simulink model "ESP_ABS"  (R2020b)
settings: Solver=VariableStepAuto  StartTime=0.0  StopTime=5  RelTol=1e-3
InitFcn:
  | ABS_F = 'ABS';
  | ABS_R = 'ABS';
  | ESP = 'ESP_moment2'
  | 
  | a = 1.203;
  | b = 1.217;
  | L = a + b;
libraries: fuzblock x5, simulink x1
settings Model: SimulationMode=accelerator  Creator=hadlaczkyb  LastModifiedBy=hadlaczkyb
settings SolverCC: AlgebraicLoopSolver=LineSearch
settings DataIOCC: ReturnWorkspaceOutputs=off
settings OptimizationCC: EfficientMapNaN2IntZero=off
settings DebuggingCC: ArithmeticOperatorsInVariantConditions=warning
settings HardwareCC: TargetBitPerPointer=64  TargetBitPerSizeT=64  TargetBitPerPtrDiffT=64  TargetLongLongMode=on  TargetIntDivRoundTo=Zero  TargetEndianess=LittleEndian  TargetWordSize=64  TargetHWDeviceType=MATLAB Host  ProdEqTarget=off
settings SFSimCC: SimUseLocalCustomCode=off  CustomCodeUndefinedFunction=UseInterfaceOnly
settings RTWCC: RTWUseLocalCustomCode=off
settings CodeAppCC: MaxIdLength=128
settings GRTTargetCC: TargetLangStandard=C89/C90 (ANSI)  CombineOutputUpdateFcns=off  GRTInterface=on

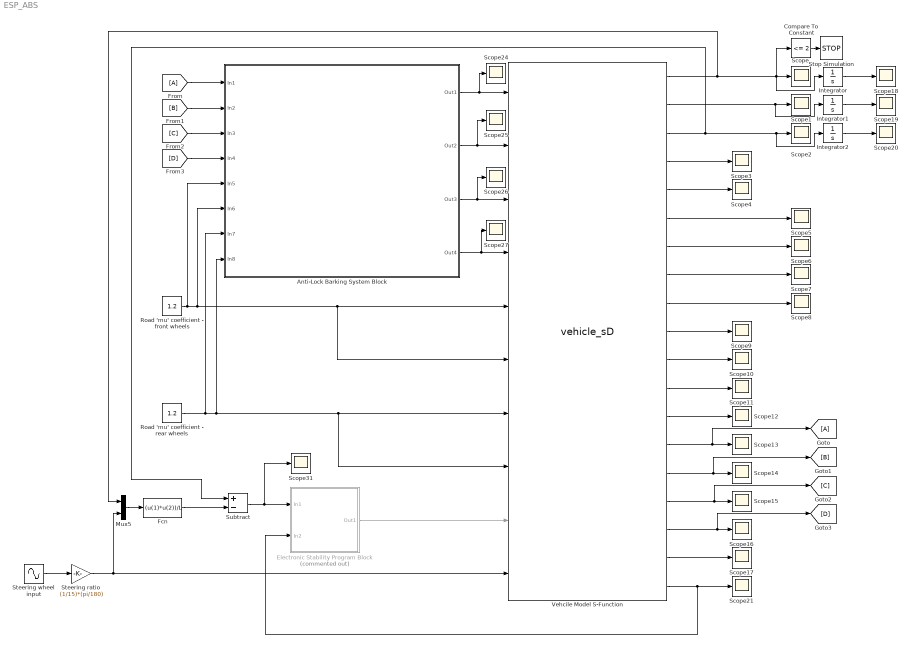
== system ESP_ABS ==
  Anti-Lock Barking System Block : Subsystem
      mask Display:
      | image('Fuzzy_ABS_ESP/ABS_icon.png');
      | port_label('input',1,'\sigma_{FL}','texmode','on');
      | port_label('input',2,'\sigma_{FR}','texmode','on');
      | port_label('input',3,'\sigma_{RL}','texmode','on');
      | port_label('input',4,'\sigma_{RR}','texmode','on');
      | port_label('input',5,'\mu_{FL}','texmode','on');
      | port_label('input',6,'\mu_{FR}','texmode','on');
      | port_label('input',7,'\mu_{RL}','texmode','on');
      | port_label('input',8,'\mu_{RR}','texmode','on');
      | port_label('output',1,'Tb_{FL}','texmode','on');
      | port_label('output',2,'Tb_{FR}','texmode','on');
      | port_label('output',3,'Tb_{RL}','texmode','on');
      | port_label('output',4,'Tb_{RR}','texmode','on');
  Compare To Constant : simulink/Logic and Bit Operations/Compare To Constant  relop=<=  const=2  OutDataTypeStr=boolean
  Electronic Stability Program Block : Subsystem  Commented=on
      mask Display:
      | image('Fuzzy_ABS_ESP/ESP_icon.png');
      | port_label('input',1,'\psi_e','texmode','on');
      | port_label('input',2,'\beta_e','texmode','on');
      | port_label('output',1,'M_z','texmode','on');
  Fcn : Fcn  Expr=(u(1)*u(2))/L
      mask Display: disp('\psi_d','texmode','on');
  Integrator : Integrator
  Integrator1 : Integrator
  Integrator2 : Integrator
  Mux5 : Mux  Inputs=2
  Road 'mu' coefficient - front wheels : Constant  Value=1.2
  Road 'mu' coefficient - rear wheels : Constant  Value=1.2
  Scope{,1..21,24..27,31} (27 alike) : Scope
  Steering ratio : Gain  Gain=(1/15)*(pi/180)
  Steering wheel input : Sin  Amplitude=0  Frequency=(2*pi)/5  SampleTime=0
  Stop Simulation : Stop
  Subtract : Sum  Inputs=+-
  Vehcile Model S-Function : M-S-Function  FunctionName=vehicle_sD
      mask Display:
      | disp('Full vehicle model');
      | port_label('input',1, 'Tb_{FL}','texmode','on');
      | port_label('input',2, 'Tb_{FR}','texmode','on');
      | port_label('input',3, 'Tb_{RL}','texmode','on');
      | port_label('input',4, 'Tb_{RR}','texmode','on');
      | port_label('input',5, '\mu_{FL}','texmode','on');
      | port_label('input',6, '\mu_{FR}','texmode','on');
      | port_label('input',7, '\mu_{RL}','texmode','on');
      | port_label('input',8, '\mu_{RR}','texmode','on');
      | port_label('input',9, 'M_z','texmode','on');
      | port_label('input',10, '\delta','texmode','on');
      | port_label('output',1,'v_{vx}','texmode','on');
      | port_label('output',2,'v_{vy}','texmode','on');
      | port_label('output',3,'\psi','texmode','on');
      | port_label('output',4,'a_{vx}','texmode','on');
      | port_label('output',5,'a_{vy}','texmode','on');
      | port_label('output',6,'v_{wxFL}','texmode','on');
      | port_label('output',7,'v_{wxFR}','texmode','on');
      | port_label('output',8,'v_{wxRL}','texmode','on');
      | port_label('output',9,'v_{wxRR}','texmode','on');
      | port_label('output',10,'\omega_{FL}','texmode','on');
      | port_label('output',11,'\omega_{FR}','texmode','on');
      | port_label('output',12,'\omega_{RL}','texmode','on');
      | port_label('output',13,'\omega_{RR}','texmode','on');
      | port_label('output',14,'\sigma_{FL}','texmode','on');
      | port_label('output',15,'\sigma_{FR}','texmode','on');
      | port_label('output',16,'\sigma_{RL}','texmode','on');
      | port_label('output',17,'\sigma_{RR}','texmode','on');
      | port_label('output',18,'v_v','texmode','on');
      | port_label('output',19,'\beta','texmode','on');
  wires:
  Vehcile Model S-Function/2 -> Integrator1/1, Scope1/1
  Vehcile Model S-Function/6 -> Scope5/1
  Vehcile Model S-Function/7 -> Scope6/1
  Vehcile Model S-Function/8 -> Scope7/1
  Vehcile Model S-Function/9 -> Scope8/1
  Vehcile Model S-Function/10 -> Scope9/1
  Vehcile Model S-Function/11 -> Scope10/1
  Vehcile Model S-Function/12 -> Scope11/1
  Vehcile Model S-Function/13 -> Scope12/1
  Vehcile Model S-Function/4 -> Scope3/1
  Vehcile Model S-Function/5 -> Scope4/1
  Integrator/1 -> Scope18/1
  Integrator1/1 -> Scope19/1
  Integrator2/1 -> Scope20/1
  Vehcile Model S-Function/18 -> Scope17/1
  Compare To Constant/1 -> Stop Simulation/1
  Fcn/1 -> Subtract/2
  Mux5/1 -> Fcn/1
  Vehcile Model S-Function/1 -> Mux5/1, Compare To Constant/1, Integrator/1, Scope/1
  Vehcile Model S-Function/15 -> [B], Scope14/1
  Vehcile Model S-Function/17 -> [D], Scope16/1
  Steering wheel input/1 -> Steering ratio/1
  Vehcile Model S-Function/3 -> Subtract/1, Scope2/1, Integrator2/1
  Vehcile Model S-Function/19 -> Electronic Stability Program Block/2(In2), Scope21/1
  Subtract/1 -> Electronic Stability Program Block/1(In1), Scope31/1
  Steering ratio/1 -> Mux5/2, Vehcile Model S-Function/10
  Anti-Lock Barking System Block/4(Out4) -> Scope27/1, Vehcile Model S-Function/4
  Anti-Lock Barking System Block/3(Out3) -> Scope26/1, Vehcile Model S-Function/3
  Anti-Lock Barking System Block/2(Out2) -> Scope25/1, Vehcile Model S-Function/2
  Anti-Lock Barking System Block/1(Out1) -> Scope24/1, Vehcile Model S-Function/1
  [A] -> Anti-Lock Barking System Block/1(In1)
  [B] -> Anti-Lock Barking System Block/2(In2)
  [C] -> Anti-Lock Barking System Block/3(In3)
  [D] -> Anti-Lock Barking System Block/4(In4)
  Electronic Stability Program Block/1(Out1) -> Vehcile Model S-Function/9
  Vehcile Model S-Function/14 -> Scope13/1, [A]
  Vehcile Model S-Function/16 -> Scope15/1, [C]
  Road 'mu' coefficient - front wheels/1 -> Anti-Lock Barking System Block/5(In5), Anti-Lock Barking System Block/6(In6), Vehcile Model S-Function/5, Vehcile Model S-Function/6
  Road 'mu' coefficient - rear wheels/1 -> Anti-Lock Barking System Block/7(In7), Anti-Lock Barking System Block/8(In8), Vehcile Model S-Function/8, Vehcile Model S-Function/7

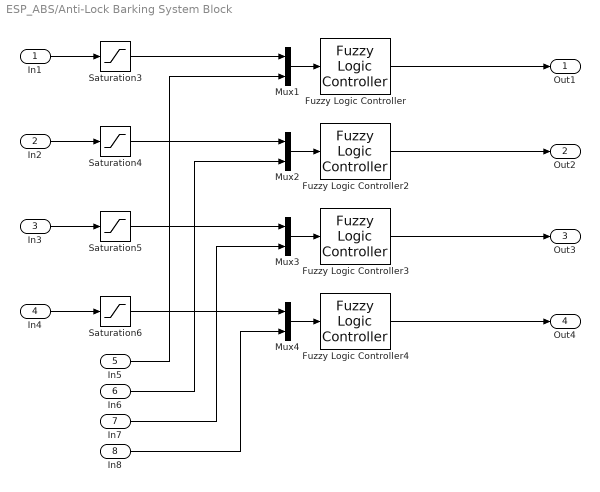
== system ESP_ABS/Anti-Lock Barking System Block ==
  In1 : Inport
  In2 : Inport  Port=2
  In3 : Inport  Port=3
  In4 : Inport  Port=4
  In5 : Inport  Port=5
  In6 : Inport  Port=6
  In7 : Inport  Port=7
  In8 : Inport  Port=8
  Fuzzy Logic Controller{,2..4} (4 alike) : fuzblock/Fuzzy Logic  Controller  FIS=ABS  OutputSampleNumber=101  DataType=double  FuzzifiedInputs=off  RuleFiringStrengths=off  RuleOutputs=off  AggregatedOutputs=off  SimulateUsing=Interpreted execution  OutOfRangeInputValueMessage=warning  NoRuleFiredMessage=warning  EmptyOutputFuzzySetMessage=warning
  Mux{1..4} (4 alike) : Mux  Inputs=2
  Saturation3 : Saturate  UpperLimit=0.15  LowerLimit=0.06
  Saturation4 : Saturate  UpperLimit=0.15  LowerLimit=0.06
  Saturation5 : Saturate  UpperLimit=0.14  LowerLimit=0.055
  Saturation6 : Saturate  UpperLimit=0.14  LowerLimit=0.055
  Out1 : Outport  VectorParamsAs1DForOutWhenUnconnected=off
  Out2 : Outport  Port=2  VectorParamsAs1DForOutWhenUnconnected=off
  Out3 : Outport  Port=3  VectorParamsAs1DForOutWhenUnconnected=off
  Out4 : Outport  Port=4  VectorParamsAs1DForOutWhenUnconnected=off
  wires:
  In3/1 -> Saturation5/1
  Mux2/1 -> Fuzzy Logic Controller2/1
  Saturation5/1 -> Mux3/1
  Mux3/1 -> Fuzzy Logic Controller3/1
  Mux4/1 -> Fuzzy Logic Controller4/1
  In1/1 -> Saturation3/1
  In2/1 -> Saturation4/1
  Saturation4/1 -> Mux2/1
  In4/1 -> Saturation6/1
  Mux1/1 -> Fuzzy Logic Controller/1
  Saturation3/1 -> Mux1/1
  Saturation6/1 -> Mux4/1
  Fuzzy Logic Controller3/1 -> Out3/1
  Fuzzy Logic Controller/1 -> Out1/1
  Fuzzy Logic Controller4/1 -> Out4/1
  Fuzzy Logic Controller2/1 -> Out2/1
  In5/1 -> Mux1/2
  In6/1 -> Mux2/2
  In7/1 -> Mux3/2
  In8/1 -> Mux4/2

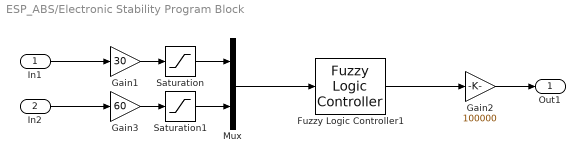
== system ESP_ABS/Electronic Stability Program Block ==
  In1 : Inport
  In2 : Inport  Port=2
  Fuzzy Logic Controller1 : fuzblock/Fuzzy Logic  Controller  FIS=ESP  OutputSampleNumber=101  DataType=double  FuzzifiedInputs=off  RuleFiringStrengths=off  RuleOutputs=off  AggregatedOutputs=off  SimulateUsing=Interpreted execution  OutOfRangeInputValueMessage=warning  NoRuleFiredMessage=warning  EmptyOutputFuzzySetMessage=warning
  Gain1 : Gain  Gain=30
  Gain2 : Gain  Gain=100000
  Gain3 : Gain  Gain=60
  Mux : Mux  Inputs=2
  Saturation : Saturate  UpperLimit=6  LowerLimit=-6
  Saturation1 : Saturate  UpperLimit=6  LowerLimit=-6
  Out1 : Outport  VectorParamsAs1DForOutWhenUnconnected=off
  wires:
  Saturation1/1 -> Mux/2
  Gain3/1 -> Saturation1/1
  Gain2/1 -> Out1/1
  Fuzzy Logic Controller1/1 -> Gain2/1
  Saturation/1 -> Mux/1
  Mux/1 -> Fuzzy Logic Controller1/1
  Gain1/1 -> Saturation/1
  In1/1 -> Gain1/1
  In2/1 -> Gain3/1
